simulink model "plant_master"  (R2019a)
settings: Solver=VariableStepAuto  StartTime=0.0  StopTime=1000  RelTol=1e-3
libraries: simulink x1
settings Model: Creator=amah2  LastModifiedBy=kovim

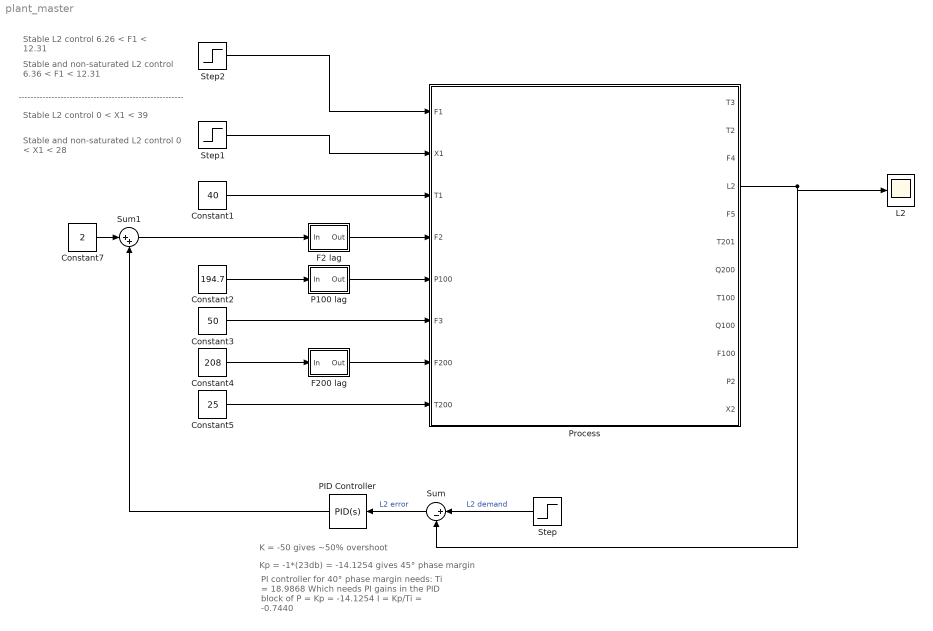
== system plant_master ==
  note: -------------------------------------------------------
  note: Stable and non-saturated L2 control
      | 6.36 < F1 < 12.31
  note: Stable L2 control
      | 6.26 < F1 < 12.31
  note: PI controller for 40° phase margin needs:
      | Ti = 18.9868
      | Which needs PI gains in the PID block of
      | P = Kp = -14.1254
      | I = Kp/Ti = -0.7440
  note: Kp = -1*(23db) = -14.1254 gives 45° phase margin
  note: K = -50 gives ~50% overshoot
  note: Stable and non-saturated L2 control
      | 0 < X1 < 28
  note: Stable L2 control
      | 0 < X1 < 39
  Constant1 : Constant  Value=40
  Constant2 : Constant  Value=194.7
  Constant3 : Constant  Value=50
  Constant4 : Constant  Value=208
  Constant5 : Constant  Value=25
  Constant7 : Constant  Value=2
  F2 lag : Subsystem
  F200 lag : Subsystem
  L2 : Scope
  P100 lag : Subsystem
  PID Controller : simulink/Continuous/PID Controller  Controller=PID  Form=Parallel  TimeDomain=Continuous-time  SampleTime=-1  IntegratorMethod=Forward Euler  FilterMethod=Forward Euler  ControllerParametersSource=internal  P=-14.1254  I=-0.7440  D=0  UseFilter=on  N=100  TunerSelectOption=Transfer Function Based (PID Tuner App)  InitialConditionSource=internal  InitialConditionForIntegrator=0  InitialConditionForFilter=0  DifferentiatorICPrevScaledInput=0  ExternalReset=none  TrackingMode=off  Kt=1  LimitOutput=off  UpperSaturationLimit=inf  LowerSaturationLimit=-inf  LinearizeAsGain=on  AntiWindupMode=none  Kb=1  POutMin=[]  POutMax=[]  IOutMin=[]  IOutMax=[]  DOutMin=[]  DOutMax=[]  NOutMin=[]  NOutMax=[]  SumOutMin=[]  SumOutMax=[]  SaturationOutMin=[]  SaturationOutMax=[]  PParamMin=[]  PParamMax=[]  IParamMin=[]  IParamMax=[]  DParamMin=[]  DParamMax=[]  NParamMin=[]  NParamMax=[]  KbParamMin=[]  KbParamMax=[]  KtParamMin=[]  KtParamMax=[]  KbOutMin=[]  KbOutMax=[]  KtOutMin=[]  KtOutMax=[]  IntegratorOutMin=[]  IntegratorOutMax=[]  FilterOutMin=[]  FilterOutMax=[]  SumI1OutMin=[]  SumI1OutMax=[]  SumI2OutMin=[]  SumI2OutMax=[]  SumI3OutMin=[]  SumI3OutMax=[]  SumI4OutMin=[]  SumI4OutMax=[]  SumDOutMin=[]  SumDOutMax=[]  DifferentiatorOutMin=[]  DifferentiatorOutMax=[]  FilterDiffOutCoefMin=[]  FilterDiffOutCoefMax=[]  ReciprocalOutMin=[]  ReciprocalOutMax=[]  SumDenOutMin=[]  SumDenOutMax=[]  SumNumOutMin=[]  SumNumOutMax=[]  DivideOutMin=[]  DivideOutMax=[]  IntegratorContinuousStateAttributes=''  IntegratorStateMustResolveToSignalObject=off  IntegratorRTWStateStorageClass=Auto  FilterContinuousStateAttributes=''  FilterStateMustResolveToSignalObject=off  FilterRTWStateStorageClass=Auto  ParallelPVariant=InternalParameters  IdealPVariant=Disabled  IVariant=InternalParameters  DVariant=InternalParameters  IntegratorVariant=Continuous  SatVariant=Disabled  AWVariant=Passthrough  PCopyVariant=Disabled  TRVariant=Disabled  FdbkBlocksVariant=Forward  IdealPFdbkVariant=Disabled  SatFdbkVariant=Disabled  DerivativeFilterVariant=ContFilter  NVariant=InternalParameters  NCopyVariant=Disabled  FilterICVariant=InternalICsFilter  IntegratorICVariant=InternalICs  ExternalResetVariant=Disabled  TRSumVariant=Passthrough  SumFdbkVariant=Disabled  SumVariant=Sum_PID
  Process : Subsystem
  Step : Step  Time=10  Before=1  SampleTime=0
  Step1 : Step  Time=10  Before=5  After=5  SampleTime=0
  Step2 : Step  Time=10  Before=10  After=6.36  SampleTime=0
  Sum : Sum  Inputs=|+-
  Sum1 : Sum  Inputs=|++
  wires:
  Process/4(L2) -> L2/1, Sum/2
  Step1/1 -> Process/2(X1)
  Constant1/1 -> Process/3(T1)
  Constant3/1 -> Process/6(F3)
  Constant4/1 -> F200 lag/1("In ")
  Constant5/1 -> Process/8(T200)
  F2 lag/1(Out) -> Process/4(F2)
  F200 lag/1(Out) -> Process/7(F200)
  Constant2/1 -> P100 lag/1("In ")
  P100 lag/1(Out) -> Process/5(P100)
  Constant7/1 -> Sum1/1
  Step/1 -> Sum/1  "L2 demand"
  Sum/1 -> PID Controller/1  "L2 error"
  PID Controller/1 -> Sum1/2
  Sum1/1 -> F2 lag/1("In ")
  Step2/1 -> Process/1(F1)

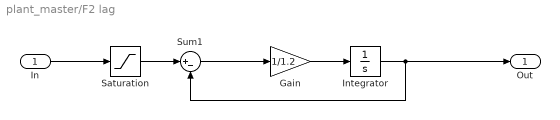
== system plant_master/F2 lag ==
  "In " : Inport
  Gain : Gain  Gain=1/1.2
  Integrator : Integrator  InitialCondition=2
  Saturation : Saturate  UpperLimit=4  LowerLimit=0
  Sum1 : Sum  Inputs=|+-
  Out : Outport
  wires:
  "In "/1 -> Saturation/1
  Sum1/1 -> Gain/1
  Gain/1 -> Integrator/1
  Integrator/1 -> Sum1/2, Out/1
  Saturation/1 -> Sum1/1

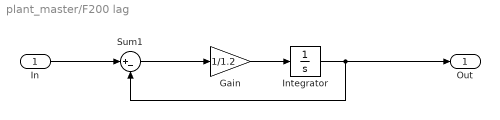
== system plant_master/F200 lag ==
  "In " : Inport
  Gain : Gain  Gain=1/1.2
  Integrator : Integrator  InitialCondition=208
  Sum1 : Sum  Inputs=|+-
  Out : Outport
  wires:
  "In "/1 -> Sum1/1
  Sum1/1 -> Gain/1
  Gain/1 -> Integrator/1
  Integrator/1 -> Sum1/2, Out/1

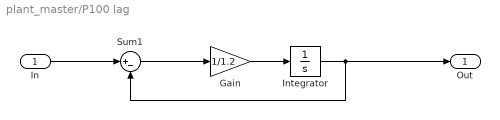
== system plant_master/P100 lag ==
  "In " : Inport
  Gain : Gain  Gain=1/1.2
  Integrator : Integrator  InitialCondition=194.7
  Sum1 : Sum  Inputs=|+-
  Out : Outport
  wires:
  "In "/1 -> Sum1/1
  Sum1/1 -> Gain/1
  Gain/1 -> Integrator/1
  Integrator/1 -> Sum1/2, Out/1

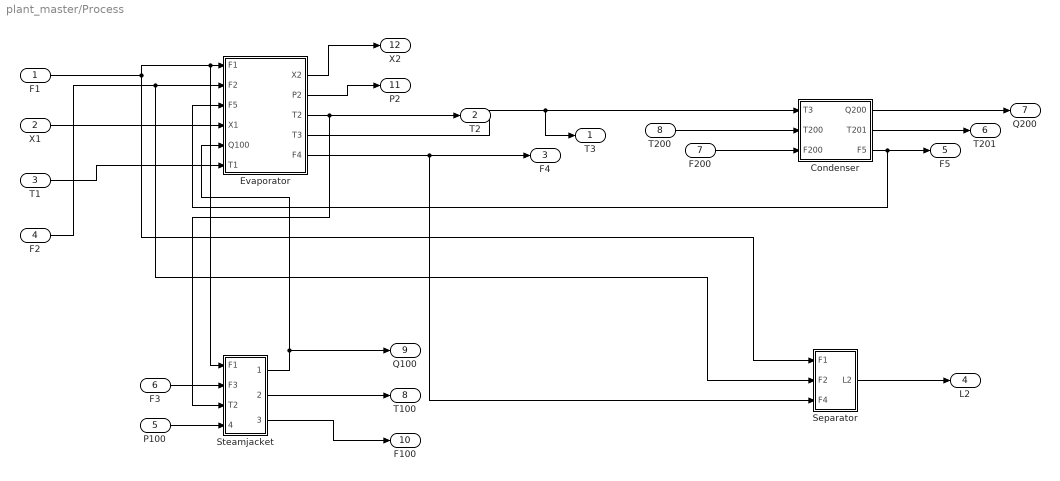
== system plant_master/Process ==
  F1 : Inport
  X1 : Inport  Port=2
  T1 : Inport  Port=3
  F2 : Inport  Port=4
  P100 : Inport  Port=5
  F3 : Inport  Port=6
  F200 : Inport  Port=7
  T200 : Inport  Port=8
  Condenser : Subsystem
  Evaporator : Subsystem
  Separator : Subsystem
  Steamjacket : Subsystem
  T3 : Outport  VectorParamsAs1DForOutWhenUnconnected=on
  T2 : Outport  Port=2  VectorParamsAs1DForOutWhenUnconnected=on
  F4 : Outport  Port=3  VectorParamsAs1DForOutWhenUnconnected=on
  L2 : Outport  Port=4  VectorParamsAs1DForOutWhenUnconnected=on
  F5 : Outport  Port=5  VectorParamsAs1DForOutWhenUnconnected=on
  T201 : Outport  Port=6  VectorParamsAs1DForOutWhenUnconnected=on
  Q200 : Outport  Port=7  VectorParamsAs1DForOutWhenUnconnected=on
  T100 : Outport  Port=8  VectorParamsAs1DForOutWhenUnconnected=on
  Q100 : Outport  Port=9  VectorParamsAs1DForOutWhenUnconnected=on
  F100 : Outport  Port=10  VectorParamsAs1DForOutWhenUnconnected=on
  P2 : Outport  Port=11  VectorParamsAs1DForOutWhenUnconnected=on
  X2 : Outport  Port=12  VectorParamsAs1DForOutWhenUnconnected=on
  wires:
  X1/1 -> Evaporator/4(X1)
  T1/1 -> Evaporator/6(T1)
  Evaporator/5("F4 ") -> F4/1, Separator/3("F4 ")
  F1/1 -> Steamjacket/1(F1), Evaporator/1(F1), Separator/1(F1)
  F2/1 -> Evaporator/2(F2), Separator/2(F2)
  F200/1 -> Condenser/3(F200)
  Evaporator/4("T3 ") -> T3/1, Condenser/1(T3)
  Evaporator/3("T2 ") -> T2/1, Steamjacket/3(T2)
  Evaporator/1(X2) -> X2/1
  Condenser/2(T201) -> T201/1
  Condenser/1(Q200) -> Q200/1
  Steamjacket/1(Q100) -> Q100/1, Evaporator/5(Q100)
  Steamjacket/2(T100) -> T100/1
  F3/1 -> Steamjacket/2(F3)
  Steamjacket/3(F100) -> F100/1
  Evaporator/2("P2 ") -> P2/1
  Separator/1(L2) -> L2/1
  Condenser/3(F5) -> F5/1, Evaporator/3(F5)
  P100/1 -> Steamjacket/4(P100)
  T200/1 -> Condenser/2(T200)

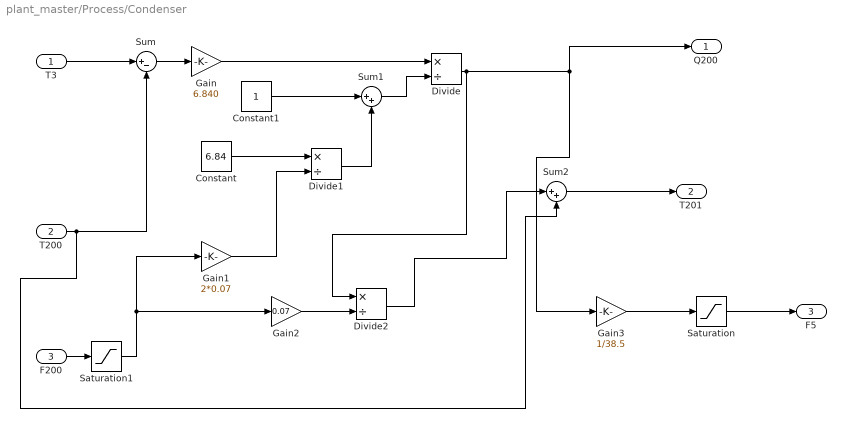
== system plant_master/Process/Condenser ==
  T3 : Inport
  T200 : Inport  Port=2
  F200 : Inport  Port=3
  Constant : Constant  Value=6.84
  Constant1 : Constant
  Divide : Product  Inputs=*/
  Divide1 : Product  Inputs=*/
  Divide2 : Product  Inputs=*/
  Gain : Gain  Gain=6.840
  Gain1 : Gain  Gain=2*0.07
  Gain2 : Gain  Gain=0.07
  Gain3 : Gain  Gain=1/38.5
  Saturation : Saturate  UpperLimit=16  LowerLimit=0
  Saturation1 : Saturate  UpperLimit=416  LowerLimit=0
  Sum : Sum  Inputs=|+-
  Sum1 : Sum  Inputs=|++
  Sum2 : Sum  Inputs=|++
  Q200 : Outport  VectorParamsAs1DForOutWhenUnconnected=on
  T201 : Outport  Port=2  VectorParamsAs1DForOutWhenUnconnected=on
  F5 : Outport  Port=3  VectorParamsAs1DForOutWhenUnconnected=on
  wires:
  Gain/1 -> Divide/1
  T200/1 -> Sum/2, Sum2/2
  T3/1 -> Sum/1
  F200/1 -> Saturation1/1
  Constant1/1 -> Sum1/1
  Sum2/1 -> T201/1
  Constant/1 -> Divide1/1
  Sum1/1 -> Divide/2
  Gain3/1 -> Saturation/1
  Divide1/1 -> Sum1/2
  Divide/1 -> Divide2/1, Q200/1, Gain3/1
  Sum/1 -> Gain/1
  Divide2/1 -> Sum2/1
  Gain2/1 -> Divide2/2
  Gain1/1 -> Divide1/2
  Saturation/1 -> F5/1
  Saturation1/1 -> Gain2/1, Gain1/1

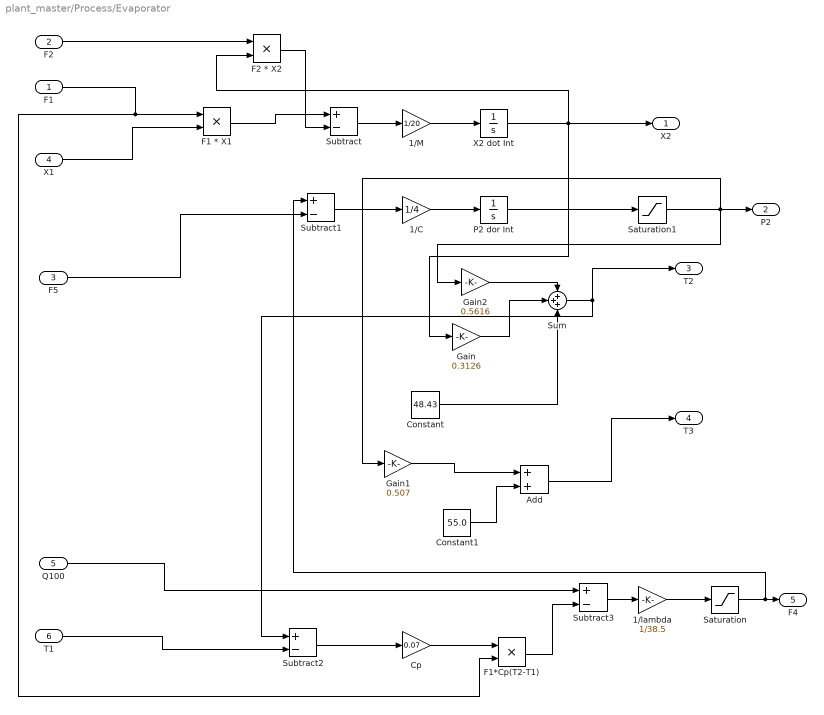
== system plant_master/Process/Evaporator ==
  F1 : Inport
  F2 : Inport  Port=2
  F5 : Inport  Port=3
  X1 : Inport  Port=4
  Q100 : Inport  Port=5
  T1 : Inport  Port=6
  1/C : Gain  Gain=1/4
  1/M : Gain  Gain=1/20
  1/lambda : Gain  Gain=1/38.5
  Add : Sum
  Constant : Constant  Value=48.43
  Constant1 : Constant  Value=55.0
  Cp : Gain  Gain=0.07
  F1 * X1 : Product
  F1*Cp(T2-T1) : Product
  F2 * X2 : Product
  Gain : Gain  Gain=0.3126
  Gain1 : Gain  Gain=0.507
  Gain2 : Gain  Gain=0.5616
  P2 dor Int : Integrator  InitialCondition=50.5
  Saturation : Saturate  UpperLimit=16  LowerLimit=0
  Saturation1 : Saturate  UpperLimit=100  LowerLimit=0
  Subtract{,1..3} (4 alike) : Sum  Inputs=+-
  Sum : Sum  Inputs=+++
  X2 dot Int : Integrator  InitialCondition=25
  X2 : Outport
  "P2 " : Outport  Port=2
  "T2 " : Outport  Port=3
  "T3 " : Outport  Port=4
  "F4 " : Outport  Port=5
  wires:
  Constant/1 -> Sum/3
  T1/1 -> Subtract2/2
  X1/1 -> F1 * X1/2
  F1*Cp(T2-T1)/1 -> Subtract3/2
  Sum/1 -> "T2 "/1, Subtract2/1
  P2 dor Int/1 -> Saturation1/1
  Constant1/1 -> Add/2
  Subtract/1 -> 1/M/1
  Subtract2/1 -> Cp/1
  1/lambda/1 -> Saturation/1
  Q100/1 -> Subtract3/1
  Cp/1 -> F1*Cp(T2-T1)/1
  Subtract1/1 -> 1/C/1
  1/C/1 -> P2 dor Int/1
  Gain2/1 -> Sum/1
  1/M/1 -> X2 dot Int/1
  F1 * X1/1 -> Subtract/1
  F2 * X2/1 -> Subtract/2
  X2 dot Int/1 -> X2/1, Gain/1, F2 * X2/2
  F2/1 -> F2 * X2/1
  Gain/1 -> Sum/2
  Add/1 -> "T3 "/1
  Gain1/1 -> Add/1
  F5/1 -> Subtract1/2
  F1/1 -> F1 * X1/1, F1*Cp(T2-T1)/2
  Subtract3/1 -> 1/lambda/1
  Saturation/1 -> "F4 "/1, Subtract1/1
  Saturation1/1 -> "P2 "/1, Gain2/1, Gain1/1

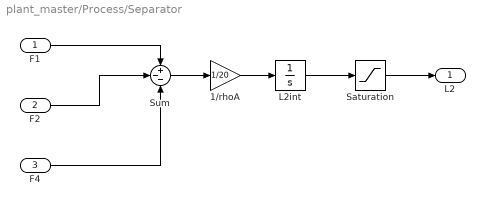
== system plant_master/Process/Separator ==
  F1 : Inport
  F2 : Inport  Port=2
  "F4 " : Inport  Port=3
  "1/rhoA " : Gain  Gain=1/20
  "L2int " : Integrator  InitialCondition=1
  Saturation : Saturate  UpperLimit=2  LowerLimit=0
  Sum : Sum  Inputs=+--
  L2 : Outport
  wires:
  "F4 "/1 -> Sum/3
  F1/1 -> Sum/1
  F2/1 -> Sum/2
  "L2int "/1 -> Saturation/1
  "1/rhoA "/1 -> "L2int "/1
  Sum/1 -> "1/rhoA "/1
  Saturation/1 -> L2/1

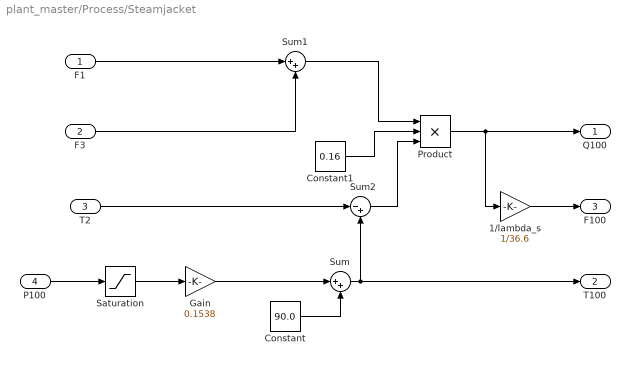
== system plant_master/Process/Steamjacket ==
  F1 : Inport
  F3 : Inport  Port=2
  T2 : Inport  Port=3
  P100 : Inport  Port=4
  1/lambda_s : Gain  Gain=1/36.6
  Constant : Constant  Value=90.0
  Constant1 : Constant  Value=0.16
  Gain : Gain  Gain=0.1538
  Product : Product  Inputs=3
  Saturation : Saturate  UpperLimit=400  LowerLimit=0
  Sum : Sum  Inputs=|++
  Sum1 : Sum  Inputs=|++
  Sum2 : Sum  Inputs=|-+
  Q100 : Outport  VectorParamsAs1DForOutWhenUnconnected=on
  T100 : Outport  Port=2  VectorParamsAs1DForOutWhenUnconnected=on
  F100 : Outport  Port=3  VectorParamsAs1DForOutWhenUnconnected=on
  wires:
  Sum/1 -> T100/1, Sum2/2
  Sum2/1 -> Product/3
  1/lambda_s/1 -> F100/1
  P100/1 -> Saturation/1
  Gain/1 -> Sum/1
  Product/1 -> Q100/1, 1/lambda_s/1
  T2/1 -> Sum2/1
  F3/1 -> Sum1/2
  Sum1/1 -> Product/1
  Constant1/1 -> Product/2
  F1/1 -> Sum1/1
  Constant/1 -> Sum/2
  Saturation/1 -> Gain/1
